simulink model "Gleichstrommaschine"  (R2022b)
settings: Solver=VariableStepAuto  StartTime=0.0  StopTime=10.0  RelTol=1e-3
values from neighbouring files (symbols this model uses):
  Cphi = 0.02    [Modell_Params.m]
  J = 10e-6    (= 1e-05)    [Modell_Params.m]
  La = 1.5e-3    (= 0.0015)    [Modell_Params.m]
  Ra = 3    [Modell_Params.m]
  Ua = 12    [Modell_Params.m]
settings Model: Creator=bornk  LastModifiedBy=bornk

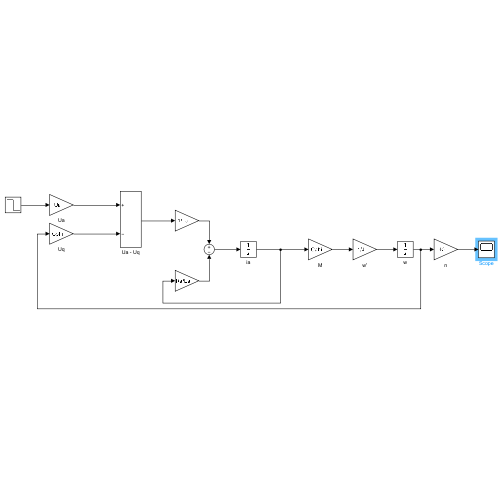
[thumbnail: Simulink's stored preview of the top-level diagram]
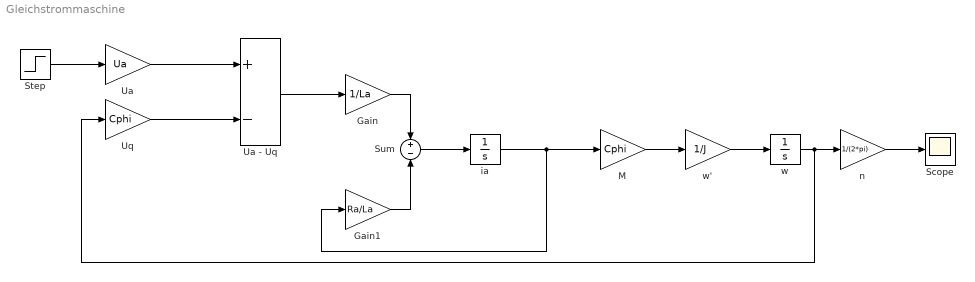
== system Gleichstrommaschine ==
  Gain : Gain  Gain=1/La
  Gain1 : Gain  Gain=Ra/La
  M : Gain  Gain=Cphi
  Scope : Scope
  Step : Step  Time=5  Before=1  After=0  SampleTime=0
  Sum : Sum  Inputs=+-
  Ua : Gain  Gain=Ua
  Ua - Uq : Sum  Inputs=+-
  Uq : Gain  Gain=Cphi
  ia : Integrator
  n : Gain  Gain=1/(2*pi)
  w : Integrator
  w' : Gain  Gain=1/J
  wires:
  Ua/1 -> Ua - Uq/1
  Uq/1 -> Ua - Uq/2
  Ua - Uq/1 -> Gain/1
  Gain/1 -> Sum/1
  Gain1/1 -> Sum/2
  Sum/1 -> ia/1
  ia/1 -> Gain1/1, M/1
  M/1 -> w'/1
  w'/1 -> w/1
  w/1 -> Uq/1, n/1
  n/1 -> Scope/1
  Step/1 -> Ua/1
